simulink model "Fig143"  (R2014a)
settings: Solver=ode3  StartTime=0  StopTime=1.0  FixedStep=1.25e-6  RelTol=1e-3
undefined symbols (not defined in the file): fdesignblkfcn, gcbh
libraries: commchan3 x1, dspvision x1
(part 2 of 2)

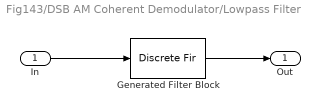
== system Fig143/DSB AM Coherent Demodulator/Lowpass Filter ==
  In : Inport
  Generated Filter Block : DiscreteFir  Tag=BlockMethodSubSystem  Coefficients=[-0.00057859688975185738 -6.35256277029553e-05 -6.6899114889850493e-05 -7.0281827960871793e-05 -7.3755351620815581e-05 -7.7281620436689229e-05 -8.0955339246433964e-05 -8.4741014547221765e-05 -8.8716681501664857e-05 -9.2804956015786759e-05 -9.7011832885440233e-05 -0.00010117277677704965 -0.00010523527131728794 -0.00010911832545827151 -0.0001132200572242036 -0.00011870380142134807 -0.0001223938337521984 -0.00012707547587606646 -0.00013168153095303027 -0.00013630632656693429 -0.00014098959404846851 -0.00014565768901793412 -0.00015036751189584986 -0.00015508317751360986 -0.00015989839112079217 -0.00016478428530502132 -0.00016977371829684953 -0.00017472486947335254 -0.00017961349729115006 -0.0001845086269574527 -0.00018981750890000542 -0.00019462827057295431 -0.00019973333272719498 -0.00020475213106112543 -0.00020981861576037196 -0.00021487383699145892 -0.00021994973669119973 -0.00022497635704710775 -0.00022998243962760856 -0.00023492996768797347 -0.00023988780074650251 -0.00024482287125012528 -0.00024973092147009709 -0.00025450987438401901 -0.00025926595722090747 -0.00026413170431046587 -0.00026875394628219002 -0.00027341954828335189 -0.00027798818353924636 -0.00028247520555216646 -0.00028690943023139794 -0.00029125831579633604 -0.00029554121694236004 -0.00029971003614987944 -0.00030378724448751923 -0.00030775923004007255 -0.0003116652784170316 -0.0003154467810397892 -0.00031907216012451239 -0.00032255402999286205 -0.00032601633826258286 -0.00032922270528635623 -0.00033237768676459671 -0.00033534831204427542 -0.00033818405667717294 -0.0003408586790543821 -0.00034339125192604157 -0.00034575833201190575 -0.00034795783281476656 -0.0003499640469809774 -0.00035179970396299312 -0.00035347126049569414 -0.00035497251683629783 -0.00035624794191293927 -0.00035732710181107411 -0.0003582645232880809 -0.00035893291678177697 -0.00035944498726020896 -0.0003597273271108813 -0.00035979667075526541 -0.00035964962004105639 -0.00035928975909587464 -0.00035872028957678311 -0.00035792796280648809 -0.0003568994240540809 -0.00035563836094284682 -0.00035416192109959273 -0.0003524639466529114 -0.00035050777285215755 -0.0003483109199713432 -0.00034591371695841488 -0.00034323152655581132 -0.00034034717782725055 -0.00033720912903652522 -0.00033382828675307456 -0.00033020084998634553 -0.0003263276821940087 -0.00032222163068519404 -0.00031787156028796946 -0.0003132742273297317 -0.0003084241982930388 -0.00030334935127542732 -0.0002980414387133588 -0.00029248546570690331 -0.00028668430648627754 -0.00028067956702794433 -0.00027440012529513224 -0.00026792603312626208 -0.00026120908684808882 -0.00025427818105373264 -0.00024711545656046051 -0.00023974055790001498 -0.00023215316921681273 -0.00022436741182116766 -0.00021636500516399672 -0.00020815930150700857 -0.00019975796547074345 -0.00019118011791842198 -0.00018240017959679673 -0.00017344473934354529 -0.00016432838728540485 -0.00015502040997375787 -0.00014556719313405946 -0.00013595528488185383 -0.00012619312289878585 -0.00011628713680748577 -0.00010623574516126244 -9.6063476140277669e-05 -8.5769623588529418e-05 -7.5363363169351529e-05 -6.4837817787230176e-05 -5.4221459480107955e-05 -4.3514878732297787e-05 -3.2720930906878138e-05 -2.1846612118911176e-05 -1.0924004427974743e-05 8.5538825744259882e-08 1.1123166178379795e-05 2.2211698185801336e-05 3.3320437333906163e-05 4.4458591148998066e-05 5.5609251002188519e-05 6.6764965200967192e-05 7.7905888116062321e-05 8.9034979293042696e-05 0.00010014143595785346 0.00011121273753790788 0.00012223133468567012 0.00013320380013046875 0.00014410680660626167 0.00015492422537374329 0.00016567393747767716 0.00017631772634519417 0.00018686143960864389 0.00019728449323855887 0.00020758396698667444 0.00021775296893650697 0.00022777618572961697 0.00023764041634039788 0.00024733948908171633 0.00025686888723354211 0.00026621289494987847 0.00027536097142532076 0.0002843143801302145 0.00029305473622739985 0.00030156487121911718 0.00030986091793204609 0.00031791055153275303 ...(+32531 chars)]  InputProcessing=Columns as channels (frame based)
  Out : Outport
  wires:
  In/1 -> Generated Filter Block/1
  Generated Filter Block/1 -> Out/1
